simulink model "L7"  (R2015a)
settings: Solver=ode45  StartTime=0.0  StopTime=10  RelTol=1e-3
libraries: dspsrcs4 x1
settings Model: Creator=User  LastModifiedBy=User

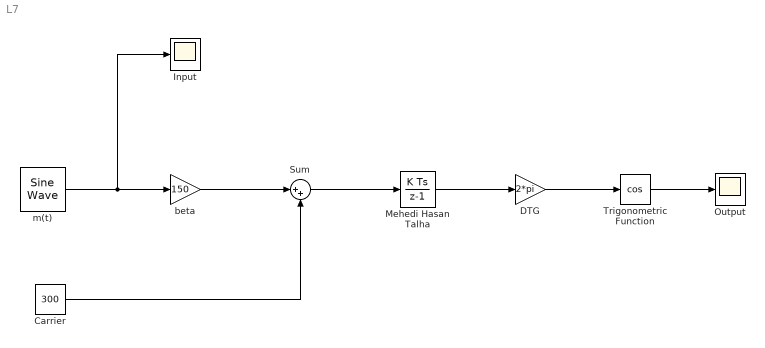
== system L7 ==
  Carrier : Constant  Value=300
  DTG : Gain  Gain=2*pi
  Input : Scope
  Mehedi Hasan Talha : DiscreteIntegrator  InitialConditionSetting=State (most efficient)  SampleTime=1/98000
  Output : Scope
      settings: SampleInput=on
  Sum : Sum  Inputs=|++
  Trigonometric Function : Trigonometry  Operator=cos
  beta : Gain  Gain=150
  m(t) : dspsrcs4/Sine Wave  Amplitude=1  Frequency=10  Phase=90  SampleMode=Discrete  OutComplex=Real  CompMethod=Trigonometric fcn  TableSize=Speed  SampleTime=1/98000  SamplesPerFrame=1  ResetState=Restart at time zero  dataType=double  wordLen=16  udDataType=sfix(16)  fracBitsMode=Best precision  numFracBits=15  OutDataTypeStr=double  LastOutDataTypeStr=double
  wires:
  m(t)/1 -> Input/1, beta/1
  beta/1 -> Sum/1
  Carrier/1 -> Sum/2
  Sum/1 -> Mehedi Hasan Talha/1
  Mehedi Hasan Talha/1 -> DTG/1
  DTG/1 -> Trigonometric Function/1
  Trigonometric Function/1 -> Output/1
